simulink model "sfcndemo_fcncallgen"  (Simulink 6.0)
settings: Solver=FixedStepDiscrete  StartTime=0.0  StopTime=10  MaxStep=0.0001  RelTol=1e-3
libraries: simulink x1
settings Model: Creator=The MathWorks Inc.  LastModifiedBy=batserve  ExtModeTrigMode=oneshot  ExtModeArmWhenConnect=off  ExtModeAutoUpdateStatusClock=off
settings DataIOCC: LimitDataPoints=off
settings OptimizationCC: BooleanDataType=off
settings DebuggingCC: CheckExecutionContextPreStartOutputMsg=on  CheckExecutionContextRuntimeOutputMsg=on  SolverPrmCheckMsg=none
settings HardwareCC: TargetUnknown=on

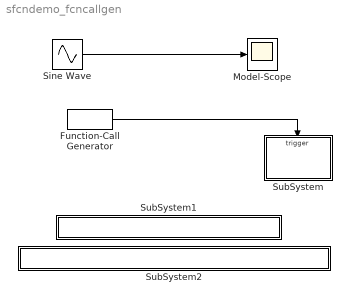
== system sfcndemo_fcncallgen ==
  Function-Call Generator : simulink/Ports & Subsystems/Function-Call Generator  sample_time=1  numberOfIterations=1
  Model-Scope : Scope
      settings: TimeRange=10
  Sine Wave : Sin  Amplitude=5  SampleTime=0.01
  SubSystem : Subsystem  PropExecContextAcrossSSBoundary=on
  SubSystem1 : Subsystem  PropExecContextAcrossSSBoundary=on
      settings: OpenFcn=edit(fullfile(matlabroot,'simulink','src','fcncallgen.c'))
      mask Display: disp('matlabroot\simulink\src\fcncallgen.c');
  SubSystem2 : Subsystem  PropExecContextAcrossSSBoundary=on
      settings: OpenFcn=edit(fullfile(matlabroot,'toolbox','simulink','blocks','tlc_c','fcncallgen.tlc'))
      mask Display: disp('matlabroot\toolbox\simulink\blocks\tlc_c\fcncallgen.tlc');
  wires:
  Sine Wave/1 -> Model-Scope/1
  Function-Call Generator/1 -> SubSystem/Trigger

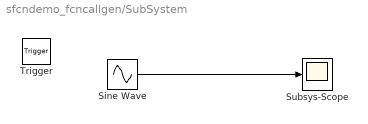
== system sfcndemo_fcncallgen/SubSystem ==
  Trigger : TriggerPort  TriggerType=function-call
  Sine Wave : Sin
  Subsys-Scope : Scope
      settings: TimeRange=10  YMin=-1  YMax=1
  wires:
  Sine Wave/1 -> Subsys-Scope/1

== system sfcndemo_fcncallgen/SubSystem1 ==

== system sfcndemo_fcncallgen/SubSystem2 ==
